simulink model "comparison"  (R2020b)
settings: Solver=VariableStepAuto  StartTime=0.0  StopTime=1.5  RelTol=1e-3
values from neighbouring files (symbols this model uses):
  A_calc = expm_taylor(Ac, T, k)    [discret_validation.m]
  A_discret = [1 T+(T^2/2)*P1 (T^2/2)*P2   (T^2/2)*P3 ... (first row only)    [discret_validation.m]
  A_ext = [1 T  (T^2)/2 0  0  0 ... (first row only)    [discret_validation.m]
  Ac = [0 1  0  0 ... (first row only)    [discret_validation.m]
  Ad = Ad + term    [discret_validation.m]
  B_discret = [(T^2/2)*P7 (T^2/2)*P8 ... (first row only)    [discret_validation.m]
  B_ext = [0  0 ... (first row only)    [discret_validation.m]
  Bc = [0  0 ... (first row only)    [discret_validation.m]
  Bd = (Ad - I) * Ac_inv * Bc    [discret_validation.m]
  T = 0.1    [discret_validation.m]
libraries: simulink_extras x1
settings Model: Creator=Admin  LastModifiedBy=Admin

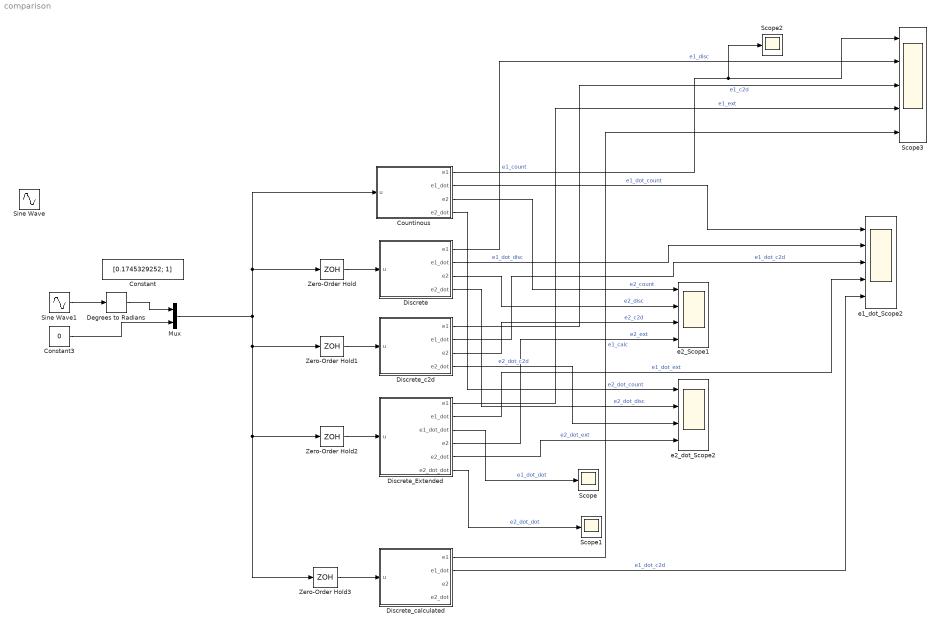
== system comparison ==
  Constant : Constant  Value=[0.1745329252; 1]
  Constant3 : Constant  Value=0
  Countinous : Subsystem
  Degrees to Radians : simulink_extras/Transformations/Degrees to Radians
  Discrete : Subsystem
  Discrete_Extended : Subsystem
  Discrete_c2d : Subsystem
  Discrete_calculated : Subsystem
  Mux : Mux  Inputs=2
  Scope : Scope
  Scope1 : Scope
  Scope2 : Scope
  Scope3 : Scope  NumInputPorts=5
  Sine Wave : Sin  Amplitude=10  SampleTime=0
  Sine Wave1 : Sin  Amplitude=3  SampleTime=0
  Zero-Order Hold{,1..3} (4 alike) : ZeroOrderHold  SampleTime=T
  e1_dot_Scope2 : Scope  NumInputPorts=5
  e2_Scope1 : Scope  NumInputPorts=4
  e2_dot_Scope2 : Scope  NumInputPorts=4
  wires:
  Zero-Order Hold/1 -> Discrete/1(u)
  Countinous/1(e1) -> Scope2/1, Scope3/1  "e1_count"
  Discrete/1(e1) -> Scope3/2  "e1_disc"
  Degrees to Radians/1 -> Mux/1
  Sine Wave1/1 -> Degrees to Radians/1
  Constant3/1 -> Mux/2
  Zero-Order Hold1/1 -> Discrete_c2d/1(u)
  Discrete_c2d/1(e1) -> Scope3/3  "e1_c2d"
  Countinous/2(e1_dot) -> e1_dot_Scope2/1  "e1_dot_count"
  Discrete/2(e1_dot) -> e1_dot_Scope2/2  "e1_dot_disc"
  Discrete_c2d/2(e1_dot) -> e1_dot_Scope2/3  "e1_dot_c2d"
  Discrete/3(e2) -> e2_Scope1/2  "e2_disc"
  Countinous/3(e2) -> e2_Scope1/1  "e2_count"
  Discrete_c2d/3(e2) -> e2_Scope1/3  "e2_c2d"
  Countinous/4(e2_dot) -> e2_dot_Scope2/1  "e2_dot_count"
  Discrete/4(e2_dot) -> e2_dot_Scope2/2  "e2_dot_disc"
  Discrete_c2d/4(e2_dot) -> e2_dot_Scope2/3  "e2_dot_c2d"
  Zero-Order Hold2/1 -> Discrete_Extended/1(u)
  Discrete_Extended/2(e1_dot) -> e1_dot_Scope2/4  "e1_dot_ext"
  Discrete_Extended/4(e2) -> e2_Scope1/4  "e2_ext"
  Discrete_Extended/5(e2_dot) -> e2_dot_Scope2/4  "e2_dot_ext"
  Discrete_Extended/3(e1_dot_dot) -> Scope/1  "e1_dot_dot"
  Discrete_Extended/6(e2_dot_dot) -> Scope1/1  "e2_dot_dot"
  Discrete_Extended/1(e1) -> Scope3/4  "e1_ext"
  Zero-Order Hold3/1 -> Discrete_calculated/1(u)
  Discrete_calculated/1(e1) -> Scope3/5  "e1_calc"
  Discrete_calculated/2(e1_dot) -> e1_dot_Scope2/5  "e1_dot_c2d"
  Mux/1 -> Zero-Order Hold3/1, Zero-Order Hold2/1, Zero-Order Hold1/1, Zero-Order Hold/1, Countinous/1(u)

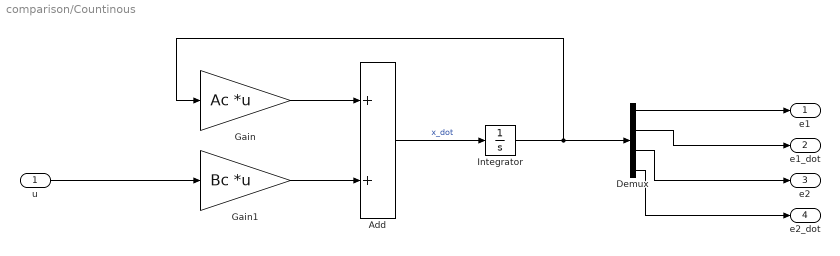
== system comparison/Countinous ==
  u : Inport
  Add : Sum
  Demux : Demux
  Gain : Gain  Gain=Ac  Multiplication=Matrix(K*u)
  Gain1 : Gain  Gain=Bc  Multiplication=Matrix(K*u)
  Integrator : Integrator
  e1 : Outport
  e1_dot : Outport  Port=2
  e2 : Outport  Port=3
  e2_dot : Outport  Port=4
  wires:
  Add/1 -> Integrator/1  "x_dot"
  Integrator/1 -> Demux/1, Gain/1
  Gain/1 -> Add/1
  Gain1/1 -> Add/2
  u/1 -> Gain1/1
  Demux/1 -> e1/1
  Demux/2 -> e1_dot/1
  Demux/3 -> e2/1
  Demux/4 -> e2_dot/1

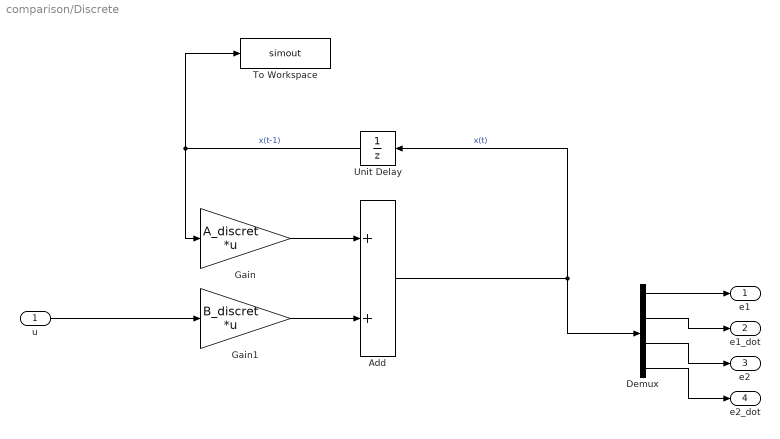
== system comparison/Discrete ==
  u : Inport
  Add : Sum
  Demux : Demux
  Gain : Gain  Gain=A_discret  Multiplication=Matrix(K*u)
  Gain1 : Gain  Gain=B_discret  Multiplication=Matrix(K*u)
  To Workspace : ToWorkspace  VariableName=simout  SaveFormat=Timeseries  SampleTime=-1
  Unit Delay : UnitDelay  SampleTime=T  HasFrameUpgradeWarning=on
  e1 : Outport
  e1_dot : Outport  Port=2
  e2 : Outport  Port=3
  e2_dot : Outport  Port=4
  wires:
  u/1 -> Gain1/1
  Gain1/1 -> Add/2
  Gain/1 -> Add/1
  Add/1 -> Unit Delay/1, Demux/1  "x(t)"
  Unit Delay/1 -> To Workspace/1, Gain/1  "x(t-1)"
  Demux/1 -> e1/1
  Demux/2 -> e1_dot/1
  Demux/3 -> e2/1
  Demux/4 -> e2_dot/1

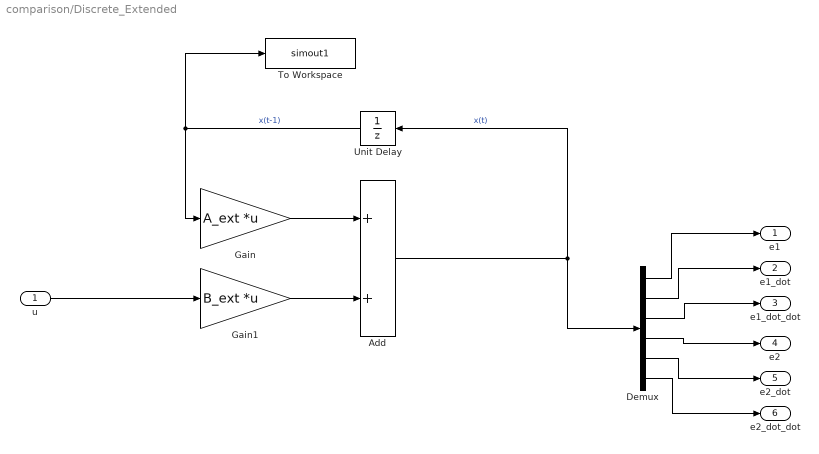
== system comparison/Discrete_Extended ==
  u : Inport
  Add : Sum
  Demux : Demux  Outputs=6
  Gain : Gain  Gain=A_ext  Multiplication=Matrix(K*u)
  Gain1 : Gain  Gain=B_ext  Multiplication=Matrix(K*u)
  To Workspace : ToWorkspace  VariableName=simout1  SaveFormat=Timeseries  SampleTime=-1
  Unit Delay : UnitDelay  SampleTime=T  HasFrameUpgradeWarning=on
  e1 : Outport
  e1_dot : Outport  Port=2
  e1_dot_dot : Outport  Port=3
  e2 : Outport  Port=4
  e2_dot : Outport  Port=5
  e2_dot_dot : Outport  Port=6
  wires:
  u/1 -> Gain1/1
  Gain1/1 -> Add/2
  Gain/1 -> Add/1
  Add/1 -> Unit Delay/1, Demux/1  "x(t)"
  Unit Delay/1 -> Gain/1, To Workspace/1  "x(t-1)"
  Demux/1 -> e1/1
  Demux/2 -> e1_dot/1
  Demux/3 -> e1_dot_dot/1
  Demux/4 -> e2/1
  Demux/5 -> e2_dot/1
  Demux/6 -> e2_dot_dot/1

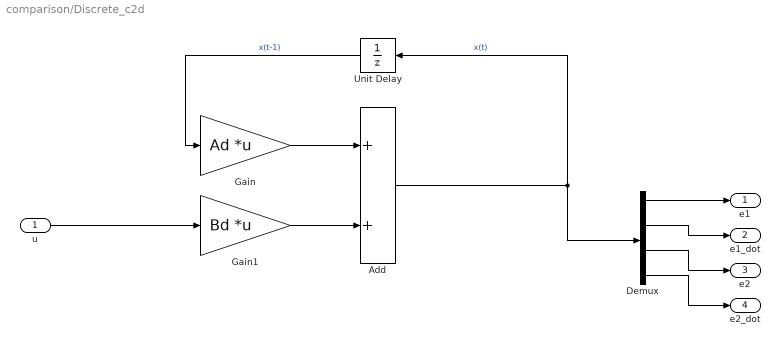
== system comparison/Discrete_c2d ==
  u : Inport
  Add : Sum
  Demux : Demux
  Gain : Gain  Gain=Ad  Multiplication=Matrix(K*u)
  Gain1 : Gain  Gain=Bd  Multiplication=Matrix(K*u)
  Unit Delay : UnitDelay  SampleTime=T  HasFrameUpgradeWarning=on
  e1 : Outport
  e1_dot : Outport  Port=2
  e2 : Outport  Port=3
  e2_dot : Outport  Port=4
  wires:
  Demux/4 -> e2_dot/1
  Demux/3 -> e2/1
  Demux/2 -> e1_dot/1
  Demux/1 -> e1/1
  Unit Delay/1 -> Gain/1  "x(t-1)"
  Add/1 -> Demux/1, Unit Delay/1  "x(t)"
  Gain/1 -> Add/1
  Gain1/1 -> Add/2
  u/1 -> Gain1/1

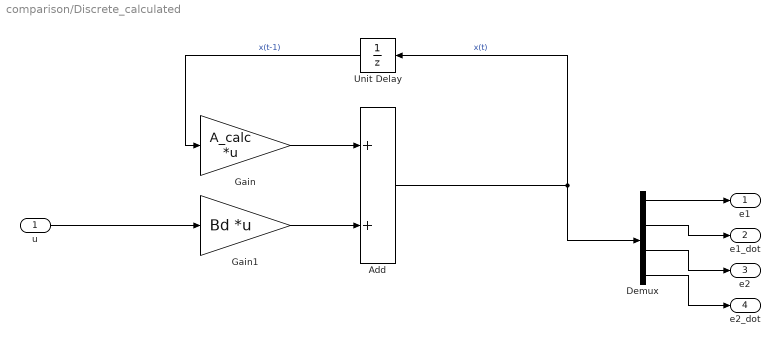
== system comparison/Discrete_calculated ==
  u : Inport
  Add : Sum
  Demux : Demux
  Gain : Gain  Gain=A_calc  Multiplication=Matrix(K*u)
  Gain1 : Gain  Gain=Bd  Multiplication=Matrix(K*u)
  Unit Delay : UnitDelay  SampleTime=T  HasFrameUpgradeWarning=on
  e1 : Outport
  e1_dot : Outport  Port=2
  e2 : Outport  Port=3
  e2_dot : Outport  Port=4
  wires:
  u/1 -> Gain1/1
  Gain1/1 -> Add/2
  Gain/1 -> Add/1
  Add/1 -> Unit Delay/1, Demux/1  "x(t)"
  Unit Delay/1 -> Gain/1  "x(t-1)"
  Demux/1 -> e1/1
  Demux/2 -> e1_dot/1
  Demux/3 -> e2/1
  Demux/4 -> e2_dot/1
